simulink model "Pose_AutoCode"  (R2019b)
settings: Solver=FixedStepDiscrete  StartTime=0.0  StopTime=10.0  RelTol=1e-3
libraries: posemodel x1

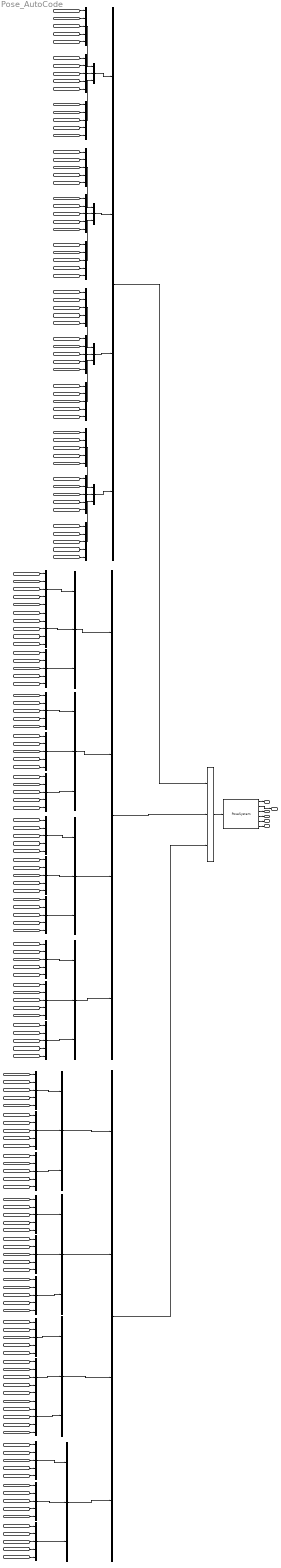
== system Pose_AutoCode ==
  accel1x_in_type : Inport  OutDataTypeStr=uint8
  accel1x_in_value : Inport  Port=2  OutDataTypeStr=double
  accel1x_in_status : Inport  Port=3  OutDataTypeStr=uint8
  accel1x_in_rms : Inport  Port=4  OutDataTypeStr=double
  accel1x_in_sequence_number : Inport  Port=5  OutDataTypeStr=uint8
  accel1y_in_type : Inport  Port=6  OutDataTypeStr=uint8
  accel1y_in_value : Inport  Port=7  OutDataTypeStr=double
  accel1y_in_status : Inport  Port=8  OutDataTypeStr=uint8
  accel1y_in_rms : Inport  Port=9  OutDataTypeStr=double
  accel1y_in_sequence_number : Inport  Port=10  OutDataTypeStr=uint8
  accel1z_in_type : Inport  Port=11  OutDataTypeStr=uint8
  accel1z_in_value : Inport  Port=12  OutDataTypeStr=double
  accel1z_in_status : Inport  Port=13  OutDataTypeStr=uint8
  accel1z_in_rms : Inport  Port=14  OutDataTypeStr=double
  accel1z_in_sequence_number : Inport  Port=15  OutDataTypeStr=uint8
  accel2x_in_type : Inport  Port=16  OutDataTypeStr=uint8
  accel2x_in_value : Inport  Port=17  OutDataTypeStr=double
  accel2x_in_status : Inport  Port=18  OutDataTypeStr=uint8
  accel2x_in_rms : Inport  Port=19  OutDataTypeStr=double
  accel2x_in_sequence_number : Inport  Port=20  OutDataTypeStr=uint8
  accel2y_in_type : Inport  Port=21  OutDataTypeStr=uint8
  accel2y_in_value : Inport  Port=22  OutDataTypeStr=double
  accel2y_in_status : Inport  Port=23  OutDataTypeStr=uint8
  accel2y_in_rms : Inport  Port=24  OutDataTypeStr=double
  accel2y_in_sequence_number : Inport  Port=25  OutDataTypeStr=uint8
  accel2z_in_type : Inport  Port=26  OutDataTypeStr=uint8
  accel2z_in_value : Inport  Port=27  OutDataTypeStr=double
  accel2z_in_status : Inport  Port=28  OutDataTypeStr=uint8
  accel2z_in_rms : Inport  Port=29  OutDataTypeStr=double
  accel2z_in_sequence_number : Inport  Port=30  OutDataTypeStr=uint8
  accel3x_in_type : Inport  Port=31  OutDataTypeStr=uint8
  accel3x_in_value : Inport  Port=32  OutDataTypeStr=double
  accel3x_in_status : Inport  Port=33  OutDataTypeStr=uint8
  accel3x_in_rms : Inport  Port=34  OutDataTypeStr=double
  accel3x_in_sequence_number : Inport  Port=35  OutDataTypeStr=uint8
  accel3y_in_type : Inport  Port=36  OutDataTypeStr=uint8
  accel3y_in_value : Inport  Port=37  OutDataTypeStr=double
  accel3y_in_status : Inport  Port=38  OutDataTypeStr=uint8
  accel3y_in_rms : Inport  Port=39  OutDataTypeStr=double
  accel3y_in_sequence_number : Inport  Port=40  OutDataTypeStr=uint8
  accel3z_in_type : Inport  Port=41  OutDataTypeStr=uint8
  accel3z_in_value : Inport  Port=42  OutDataTypeStr=double
  accel3z_in_status : Inport  Port=43  OutDataTypeStr=uint8
  accel3z_in_rms : Inport  Port=44  OutDataTypeStr=double
  accel3z_in_sequence_number : Inport  Port=45  OutDataTypeStr=uint8
  accel4x_in_type : Inport  Port=46  OutDataTypeStr=uint8
  accel4x_in_value : Inport  Port=47  OutDataTypeStr=double
  accel4x_in_status : Inport  Port=48  OutDataTypeStr=uint8
  accel4x_in_rms : Inport  Port=49  OutDataTypeStr=double
  accel4x_in_sequence_number : Inport  Port=50  OutDataTypeStr=uint8
  accel4y_in_type : Inport  Port=51  OutDataTypeStr=uint8
  accel4y_in_value : Inport  Port=52  OutDataTypeStr=double
  accel4y_in_status : Inport  Port=53  OutDataTypeStr=uint8
  accel4y_in_rms : Inport  Port=54  OutDataTypeStr=double
  accel4y_in_sequence_number : Inport  Port=55  OutDataTypeStr=uint8
  accel4z_in_type : Inport  Port=56  OutDataTypeStr=uint8
  accel4z_in_value : Inport  Port=57  OutDataTypeStr=double
  accel4z_in_status : Inport  Port=58  OutDataTypeStr=uint8
  accel4z_in_rms : Inport  Port=59  OutDataTypeStr=double
  accel4z_in_sequence_number : Inport  Port=60  OutDataTypeStr=uint8
  rotationrate1x_in_type : Inport  Port=61  OutDataTypeStr=uint8
  rotationrate1x_in_value : Inport  Port=62  OutDataTypeStr=double
  rotationrate1x_in_status : Inport  Port=63  OutDataTypeStr=uint8
  rotationrate1x_in_rms : Inport  Port=64  OutDataTypeStr=double
  rotationrate1x_in_sequence_number : Inport  Port=65  OutDataTypeStr=uint8
  rotationrate1y_in_type : Inport  Port=66  OutDataTypeStr=uint8
  rotationrate1y_in_value : Inport  Port=67  OutDataTypeStr=double
  rotationrate1y_in_status : Inport  Port=68  OutDataTypeStr=uint8
  rotationrate1y_in_rms : Inport  Port=69  OutDataTypeStr=double
  rotationrate1y_in_sequence_number : Inport  Port=70  OutDataTypeStr=uint8
  rotationrate1z_in_type : Inport  Port=71  OutDataTypeStr=uint8
  rotationrate1z_in_value : Inport  Port=72  OutDataTypeStr=double
  rotationrate1z_in_status : Inport  Port=73  OutDataTypeStr=uint8
  rotationrate1z_in_rms : Inport  Port=74  OutDataTypeStr=double
  rotationrate1z_in_sequence_number : Inport  Port=75  OutDataTypeStr=uint8
  rotationrate2x_in_type1 : Inport  Port=76  OutDataTypeStr=uint8
  rotationrate2x_in_value : Inport  Port=77  OutDataTypeStr=double
  rotationrate2x_in_status : Inport  Port=78  OutDataTypeStr=uint8
  rotationrate2x_in_rms : Inport  Port=79  OutDataTypeStr=double
  rotationrate2x_in_sequence_number : Inport  Port=80  OutDataTypeStr=uint8
  rotationrate2y_in_type : Inport  Port=81  OutDataTypeStr=uint8
  rotationrate2y_in_value : Inport  Port=82  OutDataTypeStr=double
  rotationrate2y_in_status : Inport  Port=83  OutDataTypeStr=uint8
  rotationrate2y_in_rms : Inport  Port=84  OutDataTypeStr=double
  rotationrate2y_in_sequence_number : Inport  Port=85  OutDataTypeStr=uint8
  rotationrate2z_in_type : Inport  Port=86  OutDataTypeStr=uint8
  rotationrate2z_in_value : Inport  Port=87  OutDataTypeStr=double
  rotationrate2z_in_status1 : Inport  Port=88  OutDataTypeStr=uint8
  rotationrate2z_in_rms : Inport  Port=89  OutDataTypeStr=double
  rotationrate2z_in_sequence_number : Inport  Port=90  OutDataTypeStr=uint8
  rotationrate3x_in_type : Inport  Port=91  OutDataTypeStr=uint8
  rotationrate3x_in_value : Inport  Port=92  OutDataTypeStr=double
  rotationrate3x_in_status : Inport  Port=93  OutDataTypeStr=uint8
  rotationrate3x_in_rms : Inport  Port=94  OutDataTypeStr=double
  rotationrate3x_in_sequence_number : Inport  Port=95  OutDataTypeStr=uint8
  rotationrate3y_in_type : Inport  Port=96  OutDataTypeStr=uint8
  rotationrate3y_in_value : Inport  Port=97  OutDataTypeStr=double
  rotationrate3y_in_status : Inport  Port=98  OutDataTypeStr=uint8
  rotationrate3y_in_rms : Inport  Port=99  OutDataTypeStr=double
  rotationrate3y_in_sequence_number : Inport  Port=100  OutDataTypeStr=uint8
  rotationrate3z_in_type : Inport  Port=101  OutDataTypeStr=uint8
  rotationrate3z_in_value : Inport  Port=102  OutDataTypeStr=double
  rotationrate3z_in_status : Inport  Port=103  OutDataTypeStr=uint8
  rotationrate3z_in_rms : Inport  Port=104  OutDataTypeStr=double
  rotationrate3z_in_sequence_number : Inport  Port=105  OutDataTypeStr=uint8
  rotationrate4x_in_type : Inport  Port=106  OutDataTypeStr=uint8
  rotationrate4x_in_value : Inport  Port=107  OutDataTypeStr=double
  rotationrate4x_in_status : Inport  Port=108  OutDataTypeStr=uint8
  rotationrate4x_in_rms : Inport  Port=109  OutDataTypeStr=double
  rotationrate4x_in_sequence_number : Inport  Port=110  OutDataTypeStr=uint8
  rotationrate4y_in_type : Inport  Port=111  OutDataTypeStr=uint8
  rotationrate4y_in_value : Inport  Port=112  OutDataTypeStr=double
  rotationrate4y_in_status : Inport  Port=113  OutDataTypeStr=uint8
  rotationrate4y_in_rms : Inport  Port=114  OutDataTypeStr=double
  rotationrate4y_in_sequence_number : Inport  Port=115  OutDataTypeStr=uint8
  rotationrate4z_in_type : Inport  Port=116  OutDataTypeStr=uint8
  rotationrate4z_in_value : Inport  Port=117  OutDataTypeStr=double
  rotationrate4z_in_status : Inport  Port=118  OutDataTypeStr=uint8
  rotationrate4z_in_rms : Inport  Port=119  OutDataTypeStr=double
  rotationrate4z_in_sequence_number : Inport  Port=120  OutDataTypeStr=uint8
  mag1x_in_type : Inport  Port=121  OutDataTypeStr=uint8
  mag1x_in_value : Inport  Port=122  OutDataTypeStr=double
  mag1x_in_status : Inport  Port=123  OutDataTypeStr=uint8
  mag1x_in_rms : Inport  Port=124  OutDataTypeStr=double
  mag1x_in_sequence_number : Inport  Port=125  OutDataTypeStr=uint8
  mag1y_in_type : Inport  Port=126  OutDataTypeStr=uint8
  mag1y_in_value : Inport  Port=127  OutDataTypeStr=double
  mag1y_in_status : Inport  Port=128  OutDataTypeStr=uint8
  mag1y_in_rms : Inport  Port=129  OutDataTypeStr=double
  mag1y_in_sequence_number : Inport  Port=130  OutDataTypeStr=uint8
  mag1z_in_type : Inport  Port=131  OutDataTypeStr=uint8
  mag1z_in_value : Inport  Port=132  OutDataTypeStr=double
  mag1z_in_status : Inport  Port=133  OutDataTypeStr=uint8
  mag1z_in_rms : Inport  Port=134  OutDataTypeStr=double
  mag1z_in_sequence_number : Inport  Port=135  OutDataTypeStr=uint8
  mag2x_in_type : Inport  Port=136  OutDataTypeStr=uint8
  mag2x_in_value : Inport  Port=137  OutDataTypeStr=double
  mag2x_in_status : Inport  Port=138  OutDataTypeStr=uint8
  mag2x_in_rms : Inport  Port=139  OutDataTypeStr=double
  mag2x_in_sequence_number : Inport  Port=140  OutDataTypeStr=uint8
  mag2y_in_type : Inport  Port=141  OutDataTypeStr=uint8
  mag2y_in_value : Inport  Port=142  OutDataTypeStr=double
  mag2y_in_status : Inport  Port=143  OutDataTypeStr=uint8
  mag2y_in_rms : Inport  Port=144  OutDataTypeStr=double
  mag2y_in_sequence_number : Inport  Port=145  OutDataTypeStr=uint8
  mag2z_in_type : Inport  Port=146  OutDataTypeStr=uint8
  mag2z_in_value : Inport  Port=147  OutDataTypeStr=double
  mag2z_in_status : Inport  Port=148  OutDataTypeStr=uint8
  mag2z_in_rms : Inport  Port=149  OutDataTypeStr=double
  mag2z_in_sequence_number : Inport  Port=150  OutDataTypeStr=uint8
  mag3x_in_type : Inport  Port=151  OutDataTypeStr=uint8
  mag3x_in_value : Inport  Port=152  OutDataTypeStr=double
  mag3x_in_status : Inport  Port=153  OutDataTypeStr=uint8
  mag3x_in_rms : Inport  Port=154  OutDataTypeStr=double
  mag3x_in_sequence_number : Inport  Port=155  OutDataTypeStr=uint8
  mag3y_in_type : Inport  Port=156  OutDataTypeStr=uint8
  mag3y_in_value : Inport  Port=157  OutDataTypeStr=double
  mag3y_in_status : Inport  Port=158  OutDataTypeStr=uint8
  mag3y_in_rms : Inport  Port=159  OutDataTypeStr=double
  mag3y_in_sequence_number : Inport  Port=160  OutDataTypeStr=uint8
  mag3z_in_type : Inport  Port=161  OutDataTypeStr=uint8
  mag3z_in_value : Inport  Port=162  OutDataTypeStr=double
  mag3z_in_status : Inport  Port=163  OutDataTypeStr=uint8
  mag3z_in_rms : Inport  Port=164  OutDataTypeStr=double
  mag3z_in_sequence_number : Inport  Port=165  OutDataTypeStr=uint8
  mag4x_in_type : Inport  Port=166  OutDataTypeStr=uint8
  mag4x_in_value : Inport  Port=167  OutDataTypeStr=double
  mag4x_in_status : Inport  Port=168  OutDataTypeStr=uint8
  mag4x_in_rms : Inport  Port=169  OutDataTypeStr=double
  mag4x_in_sequence_number : Inport  Port=170  OutDataTypeStr=uint8
  mag4y_in_type : Inport  Port=171  OutDataTypeStr=uint8
  mag4y_in_value : Inport  Port=172  OutDataTypeStr=double
  mag4y_in_status : Inport  Port=173  OutDataTypeStr=uint8
  mag4y_in_rms : Inport  Port=174  OutDataTypeStr=double
  mag4y_in_sequence_number : Inport  Port=175  OutDataTypeStr=uint8
  mag4z_in_type : Inport  Port=176  OutDataTypeStr=uint8
  mag4z_in_value : Inport  Port=177  OutDataTypeStr=double
  mag4z_in_status : Inport  Port=178  OutDataTypeStr=uint8
  mag4z_in_rms : Inport  Port=179  OutDataTypeStr=double
  mag4z_in_sequence_number : Inport  Port=180  OutDataTypeStr=uint8
  Bus Creator : BusCreator  Inputs=4
  Bus Creator{1,7..41} (36 alike) : BusCreator  Inputs=5
  Bus Creator{2..6,42..49} (13 alike) : BusCreator  Inputs=3
  Bus Creator50 : BusCreator  Inputs=4
  Bus Creator51 : BusCreator  Inputs=4
  PoseSystem : posemodel/PoseSystem  SystemSampleTime=-1  Latency=0  AutoFrameSizeCalculation=off
  pose_linearacceleration_signals : Outport
  Out2 : Outport  Port=2
  Out3 : Outport  Port=3
  Out4 : Outport  Port=4
  Out5 : Outport  Port=5
  Out6 : Outport  Port=6
  wires:
  PoseSystem/1 -> pose_linearacceleration_signals/1
  PoseSystem/5 -> Out2/1
  PoseSystem/3 -> Out6/1
  PoseSystem/4 -> Out3/1
  PoseSystem/6 -> Out5/1
  Bus Creator3/1 -> Bus Creator/1  "accel1_in"
  Bus Creator27/1 -> Bus Creator6/3  "accel4z_in"
  Bus Creator19/1 -> Bus Creator4/1  "accel2x_in"
  Bus Creator4/1 -> Bus Creator/2  "accel2_in"
  accel1x_in_value/1 -> Bus Creator16/2  "value"
  accel1x_in_status/1 -> Bus Creator16/3  "status"
  Bus Creator26/1 -> Bus Creator6/2  "accel4y_in"
  Bus Creator17/1 -> Bus Creator3/2  "accel1y_in"
  accel1x_in_rms/1 -> Bus Creator16/4  "rms"
  accel1y_in_value/1 -> Bus Creator17/2  "value"
  Bus Creator18/1 -> Bus Creator3/3  "accel1z_in"
  accel1y_in_type/1 -> Bus Creator17/1  "type"
  accel1z_in_value/1 -> Bus Creator18/2  "value"
  accel1z_in_rms/1 -> Bus Creator18/4  "rms"
  Bus Creator25/1 -> Bus Creator6/1  "accel4x_in"
  accel1z_in_status/1 -> Bus Creator18/3  "status"
  Bus Creator22/1 -> Bus Creator5/1  "accel3x_in"
  accel2y_in_sequence_number/1 -> Bus Creator20/5  "sequence_number"
  accel3y_in_rms/1 -> Bus Creator23/4  "rms"
  accel1x_in_type/1 -> Bus Creator16/1  "type"
  accel2z_in_type/1 -> Bus Creator21/1  "type"
  accel3y_in_value/1 -> Bus Creator23/2  "value"
  accel1y_in_sequence_number/1 -> Bus Creator17/5  "sequence_number"
  accel4x_in_status/1 -> Bus Creator25/3  "status"
  accel1y_in_rms/1 -> Bus Creator17/4  "rms"
  accel2y_in_status/1 -> Bus Creator20/3  "status"
  accel4z_in_status/1 -> Bus Creator27/3  "status"
  accel4x_in_sequence_number/1 -> Bus Creator25/5  "sequence_number"
  accel4z_in_type/1 -> Bus Creator27/1  "type"
  accel4x_in_rms/1 -> Bus Creator25/4  "rms"
  accel4y_in_rms/1 -> Bus Creator26/4  "rms"
  accel4y_in_value/1 -> Bus Creator26/2  "value"
  accel3x_in_value/1 -> Bus Creator22/2  "value"
  Bus Creator/1 -> Bus Creator2/1  "accel_in"
  accel3x_in_rms/1 -> Bus Creator22/4  "rms"
  accel3z_in_type/1 -> Bus Creator24/1  "type"
  accel3z_in_value/1 -> Bus Creator24/2  "value"
  accel2x_in_sequence_number/1 -> Bus Creator19/5  "sequence_number"
  accel2z_in_status/1 -> Bus Creator21/3  "status"
  Bus Creator24/1 -> Bus Creator5/3  "accel3z_in"
  accel3x_in_sequence_number/1 -> Bus Creator22/5  "sequence_number"
  Bus Creator23/1 -> Bus Creator5/2  "accel3y_in"
  accel2z_in_sequence_number/1 -> Bus Creator21/5  "sequence_number"
  accel4y_in_sequence_number/1 -> Bus Creator26/5  "sequence_number"
  accel4y_in_status/1 -> Bus Creator26/3  "status"
  accel1x_in_sequence_number/1 -> Bus Creator16/5  "sequence_number"
  accel1z_in_type/1 -> Bus Creator18/1  "type"
  accel2y_in_rms/1 -> Bus Creator20/4  "rms"
  accel3y_in_status/1 -> Bus Creator23/3  "status"
  accel2x_in_value/1 -> Bus Creator19/2  "value"
  Bus Creator2/1 -> PoseSystem/1  "sensor_signals"
  accel2y_in_value/1 -> Bus Creator20/2  "value"
  accel2x_in_type/1 -> Bus Creator19/1  "type"
  Bus Creator6/1 -> Bus Creator/4  "accel4_in"
  accel3y_in_sequence_number/1 -> Bus Creator23/5  "sequence_number"
  accel2x_in_rms/1 -> Bus Creator19/4  "rms"
  accel3z_in_status/1 -> Bus Creator24/3  "status"
  accel4y_in_type/1 -> Bus Creator26/1  "type"
  accel3x_in_type/1 -> Bus Creator22/1  "type"
  accel1z_in_sequence_number/1 -> Bus Creator18/5  "sequence_number"
  Bus Creator5/1 -> Bus Creator/3  "accel3_in"
  PoseSystem/2 -> Out4/1
  accel2z_in_value/1 -> Bus Creator21/2  "value"
  accel3z_in_sequence_number/1 -> Bus Creator24/5  "sequence_number"
  accel3z_in_rms/1 -> Bus Creator24/4  "rms"
  accel3y_in_type/1 -> Bus Creator23/1  "type"
  accel2x_in_status/1 -> Bus Creator19/3  "status"
  accel1y_in_status/1 -> Bus Creator17/3  "status"
  accel2z_in_rms/1 -> Bus Creator21/4  "rms"
  Bus Creator21/1 -> Bus Creator4/3  "accel2z_in"
  accel2y_in_type/1 -> Bus Creator20/1  "type"
  accel4z_in_value/1 -> Bus Creator27/2  "value"
  accel4x_in_type/1 -> Bus Creator25/1  "type"
  accel4z_in_rms/1 -> Bus Creator27/4  "rms"
  accel4x_in_value/1 -> Bus Creator25/2  "value"
  Bus Creator20/1 -> Bus Creator4/2  "accel2y_in"
  Bus Creator16/1 -> Bus Creator3/1  "accel1x_in"
  accel4z_in_sequence_number/1 -> Bus Creator27/5  "sequence_number"
  accel3x_in_status/1 -> Bus Creator22/3  "status"
  rotationrate1x_in_sequence_number/1 -> Bus Creator1/5  "sequence_number"
  rotationrate1x_in_type/1 -> Bus Creator1/1  "type"
  rotationrate1x_in_status/1 -> Bus Creator1/3  "status"
  rotationrate1x_in_value/1 -> Bus Creator1/2  "value"
  rotationrate1x_in_rms/1 -> Bus Creator1/4  "rms"
  Bus Creator1/1 -> Bus Creator42/1  "rotationrate1x_in"
  rotationrate1y_in_status/1 -> Bus Creator7/3  "status"
  Bus Creator7/1 -> Bus Creator42/2  "rotationrate1y_in"
  rotationrate1y_in_value/1 -> Bus Creator7/2  "value"
  rotationrate1y_in_type/1 -> Bus Creator7/1  "type"
  rotationrate1y_in_sequence_number/1 -> Bus Creator7/5  "sequence_number"
  rotationrate1y_in_rms/1 -> Bus Creator7/4  "rms"
  rotationrate1z_in_status/1 -> Bus Creator8/3  "status"
  Bus Creator8/1 -> Bus Creator42/3  "rotationrate1z_in"
  rotationrate1z_in_value/1 -> Bus Creator8/2  "value"
  rotationrate1z_in_type/1 -> Bus Creator8/1  "type"
  rotationrate1z_in_sequence_number/1 -> Bus Creator8/5  "sequence_number"
  rotationrate1z_in_rms/1 -> Bus Creator8/4  "rms"
  rotationrate2z_in_status1/1 -> Bus Creator11/3  "status"
  rotationrate2x_in_sequence_number/1 -> Bus Creator9/5  "sequence_number"
  rotationrate2z_in_rms/1 -> Bus Creator11/4  "rms"
  rotationrate2z_in_type/1 -> Bus Creator11/1  "type"
  Bus Creator10/1 -> Bus Creator43/2  "rotationrate2y_in"
  Bus Creator11/1 -> Bus Creator43/3  "rotationrate2z_in"
  rotationrate2y_in_type/1 -> Bus Creator10/1  "type"
  rotationrate2z_in_value/1 -> Bus Creator11/2  "value"
  rotationrate2y_in_sequence_number/1 -> Bus Creator10/5  "sequence_number"
  rotationrate2z_in_sequence_number/1 -> Bus Creator11/5  "sequence_number"
  rotationrate2x_in_type1/1 -> Bus Creator9/1  "type"
  rotationrate2x_in_value/1 -> Bus Creator9/2  "value"
  Bus Creator9/1 -> Bus Creator43/1  "rotationrate2x_in"
  rotationrate2x_in_status/1 -> Bus Creator9/3  "status"
  rotationrate2x_in_rms/1 -> Bus Creator9/4  "rms"
  rotationrate2y_in_value/1 -> Bus Creator10/2  "value"
  rotationrate2y_in_status/1 -> Bus Creator10/3  "status"
  rotationrate2y_in_rms/1 -> Bus Creator10/4  "rms"
  rotationrate3z_in_status/1 -> Bus Creator14/3  "status"
  rotationrate3x_in_sequence_number/1 -> Bus Creator12/5  "sequence_number"
  rotationrate3z_in_rms/1 -> Bus Creator14/4  "rms"
  rotationrate3z_in_type/1 -> Bus Creator14/1  "type"
  Bus Creator13/1 -> Bus Creator44/2  "rotationrate3y_in"
  Bus Creator14/1 -> Bus Creator44/3  "rotationrate3z_in"
  rotationrate3y_in_type/1 -> Bus Creator13/1  "type"
  rotationrate3z_in_value/1 -> Bus Creator14/2  "value"
  rotationrate3y_in_sequence_number/1 -> Bus Creator13/5  "sequence_number"
  rotationrate3z_in_sequence_number/1 -> Bus Creator14/5  "sequence_number"
  rotationrate3x_in_type/1 -> Bus Creator12/1  "type"
  rotationrate3x_in_value/1 -> Bus Creator12/2  "value"
  Bus Creator12/1 -> Bus Creator44/1  "rotationrate3x_in"
  rotationrate3x_in_status/1 -> Bus Creator12/3  "status"
  rotationrate3x_in_rms/1 -> Bus Creator12/4  "rms"
  rotationrate3y_in_value/1 -> Bus Creator13/2  "value"
  rotationrate3y_in_status/1 -> Bus Creator13/3  "status"
  rotationrate3y_in_rms/1 -> Bus Creator13/4  "rms"
  rotationrate4z_in_status/1 -> Bus Creator29/3  "status"
  rotationrate4x_in_sequence_number/1 -> Bus Creator15/5  "sequence_number"
  rotationrate4z_in_rms/1 -> Bus Creator29/4  "rms"
  rotationrate4z_in_type/1 -> Bus Creator29/1  "type"
  Bus Creator28/1 -> Bus Creator45/2  "rotationrate4y_in"
  Bus Creator29/1 -> Bus Creator45/3  "rotationrate4z_in"
  rotationrate4y_in_type/1 -> Bus Creator28/1  "type"
  rotationrate4z_in_value/1 -> Bus Creator29/2  "value"
  rotationrate4y_in_sequence_number/1 -> Bus Creator28/5  "sequence_number"
  rotationrate4z_in_sequence_number/1 -> Bus Creator29/5  "sequence_number"
  rotationrate4x_in_type/1 -> Bus Creator15/1  "type"
  rotationrate4x_in_value/1 -> Bus Creator15/2  "value"
  Bus Creator15/1 -> Bus Creator45/1  "rotationrate4x_in"
  rotationrate4x_in_status/1 -> Bus Creator15/3  "status"
  rotationrate4x_in_rms/1 -> Bus Creator15/4  "rms"
  rotationrate4y_in_value/1 -> Bus Creator28/2  "value"
  rotationrate4y_in_status/1 -> Bus Creator28/3  "status"
  rotationrate4y_in_rms/1 -> Bus Creator28/4  "rms"
  mag1x_in_status/1 -> Bus Creator30/3  "status"
  Bus Creator30/1 -> Bus Creator46/1  "mag1x_in"
  mag1x_in_value/1 -> Bus Creator30/2  "value"
  mag1x_in_type/1 -> Bus Creator30/1  "type"
  mag1x_in_sequence_number/1 -> Bus Creator30/5  "sequence_number"
  mag1x_in_rms/1 -> Bus Creator30/4  "rms"
  mag1y_in_value/1 -> Bus Creator31/2  "value"
  mag1y_in_type/1 -> Bus Creator31/1  "type"
  mag1y_in_status/1 -> Bus Creator31/3  "status"
  Bus Creator31/1 -> Bus Creator46/2  "mag1y_in"
  mag1y_in_sequence_number/1 -> Bus Creator31/5  "sequence_number"
  mag1y_in_rms/1 -> Bus Creator31/4  "rms"
  mag1z_in_value/1 -> Bus Creator32/2  "value"
  mag1z_in_type/1 -> Bus Creator32/1  "type"
  mag1z_in_status/1 -> Bus Creator32/3  "status"
  Bus Creator32/1 -> Bus Creator46/3  "mag1z_in"
  mag1z_in_sequence_number/1 -> Bus Creator32/5  "sequence_number"
  mag1z_in_rms/1 -> Bus Creator32/4  "rms"
  mag2z_in_value/1 -> Bus Creator35/2  "value"
  mag2x_in_rms/1 -> Bus Creator33/4  "rms"
  mag2z_in_status/1 -> Bus Creator35/3  "status"
  mag2y_in_value/1 -> Bus Creator34/2  "value"
  mag2y_in_rms/1 -> Bus Creator34/4  "rms"
  Bus Creator35/1 -> Bus Creator47/3  "mag2z_in"
  mag2y_in_sequence_number/1 -> Bus Creator34/5  "sequence_number"
  mag2x_in_status/1 -> Bus Creator33/3  "status"
  mag2y_in_type/1 -> Bus Creator34/1  "type"
  mag2x_in_type/1 -> Bus Creator33/1  "type"
  mag2z_in_rms/1 -> Bus Creator35/4  "rms"
  mag2y_in_status/1 -> Bus Creator34/3  "status"
  mag2x_in_value/1 -> Bus Creator33/2  "value"
  mag2x_in_sequence_number/1 -> Bus Creator33/5  "sequence_number"
  Bus Creator34/1 -> Bus Creator47/2  "mag2y_in"
  mag2z_in_type/1 -> Bus Creator35/1  "type"
  mag2z_in_sequence_number/1 -> Bus Creator35/5  "sequence_number"
  Bus Creator33/1 -> Bus Creator47/1  "mag2x_in"
  mag3z_in_value/1 -> Bus Creator38/2  "value"
  mag3x_in_rms/1 -> Bus Creator36/4  "rms"
  mag3z_in_status/1 -> Bus Creator38/3  "status"
  mag3y_in_value/1 -> Bus Creator37/2  "value"
  mag3y_in_rms/1 -> Bus Creator37/4  "rms"
  Bus Creator38/1 -> Bus Creator48/3  "mag3z_in"
  mag3y_in_sequence_number/1 -> Bus Creator37/5  "sequence_number"
  mag3x_in_status/1 -> Bus Creator36/3  "status"
  mag3y_in_type/1 -> Bus Creator37/1  "type"
  mag3x_in_type/1 -> Bus Creator36/1  "type"
  mag3z_in_rms/1 -> Bus Creator38/4  "rms"
  mag3y_in_status/1 -> Bus Creator37/3  "status"
  mag3x_in_value/1 -> Bus Creator36/2  "value"
  mag3x_in_sequence_number/1 -> Bus Creator36/5  "sequence_number"
  Bus Creator37/1 -> Bus Creator48/2  "mag3y_in"
  mag3z_in_type/1 -> Bus Creator38/1  "type"
  mag3z_in_sequence_number/1 -> Bus Creator38/5  "sequence_number"
  Bus Creator36/1 -> Bus Creator48/1  "mag3x_in"
  mag4z_in_value/1 -> Bus Creator41/2  "value"
  mag4x_in_rms/1 -> Bus Creator39/4  "rms"
  mag4z_in_status/1 -> Bus Creator41/3  "status"
  mag4y_in_value/1 -> Bus Creator40/2  "value"
  mag4y_in_rms/1 -> Bus Creator40/4  "rms"
  Bus Creator41/1 -> Bus Creator49/3  "mag4z_in"
  mag4y_in_sequence_number/1 -> Bus Creator40/5  "sequence_number"
  mag4x_in_status/1 -> Bus Creator39/3  "status"
  mag4y_in_type/1 -> Bus Creator40/1  "type"
  mag4x_in_type/1 -> Bus Creator39/1  "type"
  mag4z_in_rms/1 -> Bus Creator41/4  "rms"
  mag4y_in_status/1 -> Bus Creator40/3  "status"
  mag4x_in_value/1 -> Bus Creator39/2  "value"
  mag4x_in_sequence_number/1 -> Bus Creator39/5  "sequence_number"
  Bus Creator40/1 -> Bus Creator49/2  "mag4y_in"
  mag4z_in_type/1 -> Bus Creator41/1  "type"
  mag4z_in_sequence_number/1 -> Bus Creator41/5  "sequence_number"
  Bus Creator39/1 -> Bus Creator49/1  "mag4x_in"
  Bus Creator42/1 -> Bus Creator50/1  "rotationrate1_in"
  Bus Creator43/1 -> Bus Creator50/2  "rotationrate2_in"
  Bus Creator44/1 -> Bus Creator50/3  "rotationrate3_in"
  Bus Creator45/1 -> Bus Creator50/4  "rotationrate4_in"
  Bus Creator46/1 -> Bus Creator51/1  "mag1_in"
  Bus Creator47/1 -> Bus Creator51/2  "mag2_in"
  Bus Creator48/1 -> Bus Creator51/3  "mag3_in"
  Bus Creator49/1 -> Bus Creator51/4  "mag4_in"
  Bus Creator50/1 -> Bus Creator2/2  "rotationrate_in"
  Bus Creator51/1 -> Bus Creator2/3  "mag_in"
